simulink model "SVD_Ex1"  (R2025a)
settings: Solver=VariableStepAuto  StartTime=0.0  StopTime=10  RelTol=1e-3
undefined symbols (not defined in the file): S, static_input_Convolution_Stream_Ex1, Subsystem, vsva2197, xcvc1902
libraries: aieUtilities x3, matrix_library x2, aieSolver x1, vmcUtilities x1
settings Model: Creator=sdegala  LastModifiedBy=sdegala
settings ModelReferenceCC: EnableRefExpFcnMdlSchedulingChecks=on
settings RTWCC: GPUComputeCapability=3.5

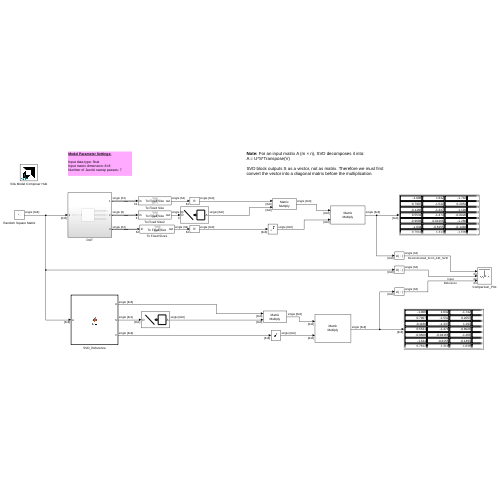
[thumbnail: Simulink's stored preview of the top-level diagram]
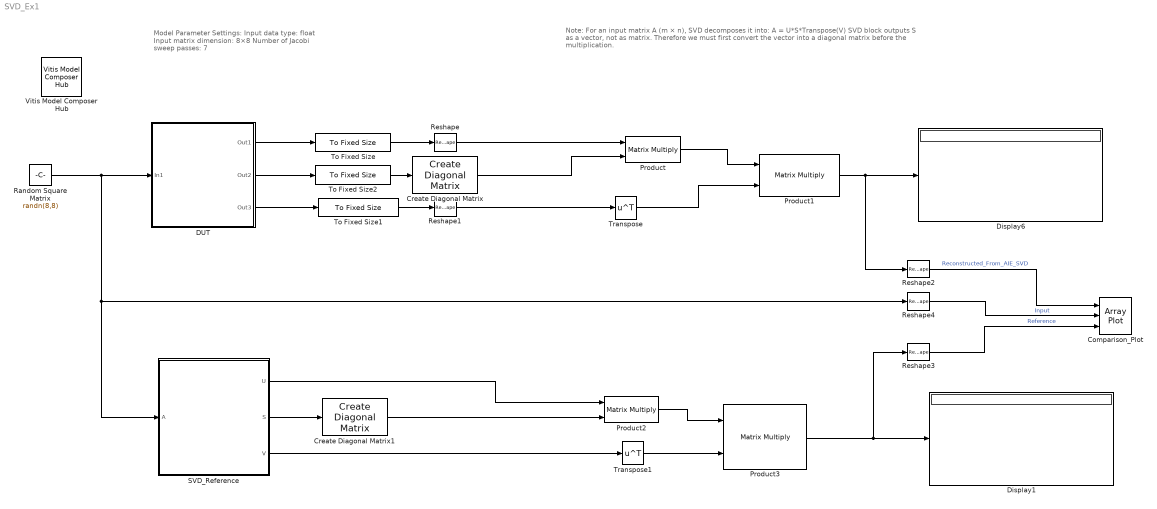
== system SVD_Ex1 ==
  note: Note: For an input matrix A (m × n), SVD decomposes it into:
      | A = U*S*Transpose(V)
      |
      | SVD block outputs S as a vector, not as matrix. Therefore we must first convert the vector into a diagonal matrix before the multiplication.
  note: Model Parameter Settings:
      |
      | Input data type: float
      | Input matrix dimension: 8×8
      | Number of Jacobi sweep passes: 7
  Comparison_Plot : ArrayPlot  NumInputPorts=3  WindowPosition=[560.000000,350.000000,800.000000,500.000000,]  Visible=on  ScopeFrameLocation=window  YLimits=[-2.5086 2.2938]  ShowLegend=on
  Create Diagonal Matrix : matrix_library/Create Diagonal Matrix
      settings: LibrarySourceBlock=|
      | simulink/Matrix
      | Operations/Create Diagonal
      | Matrix
  Create Diagonal Matrix1 : matrix_library/Create Diagonal Matrix
      settings: LibrarySourceBlock=|
      | simulink/Matrix
      | Operations/Create Diagonal
      | Matrix
  DUT : Subsystem
  Display1 : Display
  Display6 : Display
  Product{,1..3} (4 alike) : Product  Multiplication=Matrix(*)
  Random Square Matrix : Constant  Value=randn(8,8)  OutDataTypeStr=single  SampleTime=1
  Reshape : Reshape  OutputDimensionality=Customize  OutputDimensions=[8,8]
  Reshape1 : Reshape  OutputDimensionality=Customize  OutputDimensions=[8,8]
  Reshape2 : Reshape
  Reshape3 : Reshape
  Reshape4 : Reshape
  SVD_Reference : MATLAB Function  TreatAsAtomicUnit=on
  To Fixed Size : aieUtilities/To Fixed Size  Mode=Stop simulation when input variable-size signal is not full  OutputSize=Inherit: Same as input  CopyMethod=Buffer samples to form output  HasStatusOutput=on
  To Fixed Size1 : aieUtilities/To Fixed Size  Mode=Stop simulation when input variable-size signal is not full  OutputSize=Inherit: Same as input  CopyMethod=Buffer samples to form output  HasStatusOutput=on
  To Fixed Size2 : aieUtilities/To Fixed Size  Mode=Stop simulation when input variable-size signal is not full  OutputSize=Inherit: Same as input  CopyMethod=Buffer samples to form output  HasStatusOutput=on
  Transpose : Math  Operator=transpose
  Transpose1 : Math  Operator=transpose
  Vitis Model Composer Hub : vmcUtilities/Vitis Model Composer Hub  Tag=genX  CodeGeneration=off  SubsystemName=Subsystem  BlockHierPath=static_input_Convolution_Stream_Ex1/Subsystem  SubsystemType=AIENode  AIEArrayConfig=Use entire AIE array  StartColumn=1  NumberOfColumns=1  TargetDirectory=./code  exportDesign=on  analyzeDesign=off  validateDesignOnHw=off  ExportType=AI Engines  IpVendor=xilinx.com  IpLibrary=hls  IpVersion=1.0  IpHWLanguage=Verilog  AieCompilerOptions={}  AieSimulatorOptions={}  CreateTestbench=on  TestbenchStackSize=10  RunRtlSim=off  RunCSim=off  RunAieSim=off  enableSimulationTimeout=on  enableGraphIterations=on  AieSimTimeout=50000  AieGraphIterations=-1  RunAieSimProfiling=off  LaunchVitisAnalyzer=off  PlotOutput=off  RunX86Sim=off  X86SimTimeout=10  GenHwImage=off  GenLibadfXo=off  GenHwValidationCode=off  PlatformType=Not Specified  HwSystemType=Baremetal  HwValidationTarget=hw  ProjDevice=xcvc1902-vsva2197-1LP-e-S  ProjDevicePart=xcvc1902-vsva2197-1LP-e-S  AIEType=AIE  SamplePeriod=-1  ClockFrequency=200  DataPathParallelism=1  xilinxfamily=versalaicore  part=xcvc1902  speed=-1LP-e-S  package=vsva2197  directory=./netlist  testbench=off  incr_netlist=off  synthesis_tool=Vivado  clock_wrapper=Clock Enables  dbl_ovrd=According to Block Masks  dcm_input_clock_period=10  sysclk_period=10  simulink_period=1  eval_field=0  IPInfoJsonString="{\"DUTSubsystemName\":\"Subsystem\",\"AIESubsystem\":{\"SubsystemName\":\"Subsystem\",\"TargetDirectory\":\"./code\",\"AIEArrayConfig\":\"Use entire AIE array\",\"StartColumn\":\"0\",\"NumberOfColumns\":\"1\"},\"SubsystemTag\":\"AIENode\"}"  LogFileName=/tmp/CR-1250814/code/model_composer.log  NThreads=4  IPConfigFile=/tmp/vmctmp-13380004059271250980/static_input_Convolution_Stream_Ex1_ipconfig.json
  wires:
  SVD_Reference/2(S) -> Create Diagonal Matrix1/1
  Reshape/1 -> Product/1
  Reshape1/1 -> Transpose/1
  To Fixed Size/1 -> Reshape/1
  To Fixed Size1/1 -> Reshape1/1
  To Fixed Size2/1 -> Create Diagonal Matrix/1
  Product1/1 -> Reshape2/1, Display6/1
  Product/1 -> Product1/1
  Transpose/1 -> Product1/2
  Create Diagonal Matrix/1 -> Product/2
  DUT/1(Out1) -> To Fixed Size/1
  DUT/2(Out2) -> To Fixed Size2/1
  DUT/3(Out3) -> To Fixed Size1/1
  Transpose1/1 -> Product3/2
  Create Diagonal Matrix1/1 -> Product2/2
  SVD_Reference/1(U) -> Product2/1
  SVD_Reference/3(V) -> Transpose1/1
  Product2/1 -> Product3/1
  Product3/1 -> Reshape3/1, Display1/1
  Reshape2/1 -> Comparison_Plot/1  "Reconstructed_From_AIE_SVD"
  Reshape3/1 -> Comparison_Plot/3  "Reference"
  Random Square Matrix/1 -> DUT/1(In1), Reshape4/1, SVD_Reference/1(A)
  Reshape4/1 -> Comparison_Plot/2  "Input"

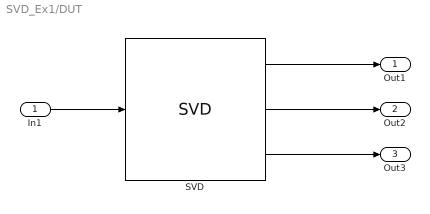
== system SVD_Ex1/DUT ==
  In1 : Inport
  SVD : aieSolver/SVD  AIE_VARIANT=1  data_type=float  row_dimension=8  cols_dimension=8  num_passes=7  casc_length=1  blockJsonConstraints=[]  blockJsonConstraintsInternal=[]  spec=vmc_svd.json  SerializedMaskParamNames=[]  SerializedMaskParamValues=[]  SerializedMaskParamVisibilities=[]  block_type=SVD  SerializedMaskParamDataypes=uint|typename|uint|uint|uint|uint  SerializedMaskParamEnumStrArr=0|0|0|0|0|0  SerializedMaskParamEnumValArr=0|0|0|0|0|0  SerializedMaskParamVectorArr=0|0|0|0|0|0  SerializedMaskParamKeys=AIE_VARIANT|TT_DATA|TP_DIM_ROWS|TP_DIM_COLS|TP_PASSES|TP_CASC_LEN
  Out1 : Outport
  Out2 : Outport  Port=2
  Out3 : Outport  Port=3
  wires:
  SVD/3 -> Out3/1
  SVD/1 -> Out1/1
  SVD/2 -> Out2/1
  In1/1 -> SVD/1

== matlab function SVD_Ex1/SVD_Reference ==
  data: A input; U output; S output; V output
function [U,S,V] = fcn(A)

[U,S,V] = svd(A,"econ","vector");
